simulink subsystem "aerodynamics_subsystem"  (R2025a)
settings: Solver=VariableStepAuto  StartTime=0.0  StopTime=10.0  RelTol=1e-3
values from neighbouring files (symbols this model uses):
  aero_surf = 0.2    [actual_uav_parameters_xflr5.m]
  aoa_rad = (aoa_degree*pi)/180    [actual_uav_parameters_xflr5.m]
  Cd = [0.027107 ... (first row only)    [actual_uav_parameters_xflr5.m]
  Cl = [-0.11803 ... (first row only)    [actual_uav_parameters_xflr5.m]
settings Model: Creator=Zyad  LastModifiedBy=Zyad

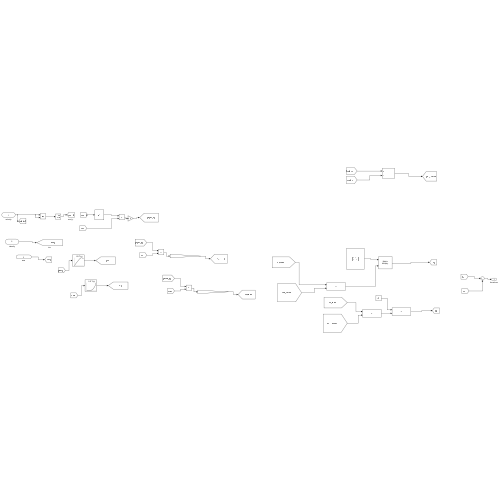
[thumbnail: Simulink's stored preview of the top-level diagram]
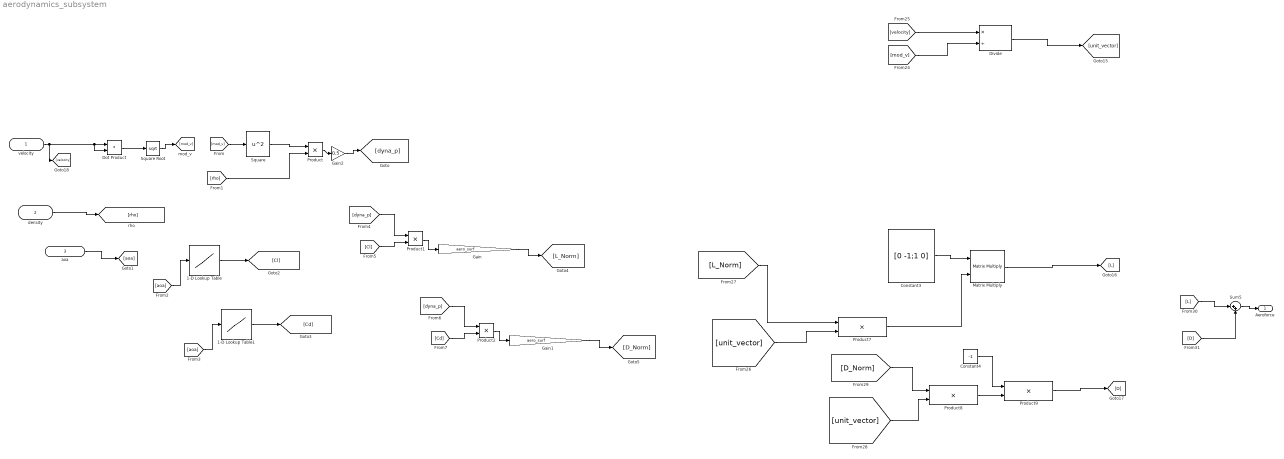
== system aerodynamics_subsystem ==
  velocity : Inport
  density : Inport  Port=2
  aoa : Inport  Port=3
  1-D Lookup Table : Lookup_n-D  NumberOfTableDimensions=1  BreakpointsForDimension1=aoa_rad  Table=Cl  InternalRulePriority=Speed  RndMeth=Simplest
  1-D Lookup Table1 : Lookup_n-D  NumberOfTableDimensions=1  BreakpointsForDimension1=aoa_rad  Table=Cd  InternalRulePriority=Speed  RndMeth=Simplest
  Constant3 : Constant  Value=[0 -1;1 0]
  Constant4 : Constant  Value=-1
  Divide : Product  Inputs=*/
  Dot Product : DotProduct  OutDataTypeStr=Inherit: Inherit via internal rule
  Gain : Gain  Gain=aero_surf
  Gain1 : Gain  Gain=aero_surf
  Gain2 : Gain  Gain=0.5
  Matrix Multiply : Product  Multiplication=Matrix(*)
  Product{,1..2,7..9} (6 alike) : Product
  Square : Math  Operator=square
  Square Root : Sqrt
  Sum5 : Sum  Inputs=|++
  Aeroforce : Outport
  wires:
  velocity/1 -> Dot Product/2, Dot Product/1, [velocity]
  Dot Product/1 -> Square Root/1
  Square Root/1 -> [mod_v]
  density/1 -> [rho]
  [mod_v] -> Square/1
  [rho] -> Product/2
  Square/1 -> Product/1
  aoa/1 -> [aoa]
  [aoa] -> 1-D Lookup Table/1
  1-D Lookup Table/1 -> [Cl]
  [aoa] -> 1-D Lookup Table1/1
  1-D Lookup Table1/1 -> [Cd]
  [dyna_p] -> Product1/1
  [Cl] -> Product1/2
  Product1/1 -> Gain/1
  Gain/1 -> [L_Norm]
  [dyna_p] -> Product2/1
  Product2/1 -> Gain1/1
  [Cd] -> Product2/2
  Gain1/1 -> [D_Norm]
  Divide/1 -> [unit_vector]
  [L_Norm] -> Product7/1
  [unit_vector] -> Product7/2
  [unit_vector] -> Product8/2
  [D_Norm] -> Product8/1
  Product8/1 -> Product9/2
  Constant4/1 -> Product9/1
  Product7/1 -> Matrix Multiply/2
  Constant3/1 -> Matrix Multiply/1
  Matrix Multiply/1 -> [L]
  Product9/1 -> [D]
  [D] -> Sum5/2
  [L] -> Sum5/1
  Sum5/1 -> Aeroforce/1
  Product/1 -> Gain2/1
  Gain2/1 -> [dyna_p]
  [velocity] -> Divide/1
  [mod_v] -> Divide/2
